simulink library "Wheels_Driver_VehDyn_Lib"  (R2018a)
settings: Solver=VariableStepAuto  StartTime=0.0  StopTime=10.0  RelTol=1e-3
undefined symbols (not defined in the file): I, Kbr, P, vehicleMass
libraries: autolibshared x3, simulink x1
(part 1 of 3)
settings Model: Creator=emarquez  LastModifiedBy=emarquez
settings CodeAppCC: StateflowObjectComments=on

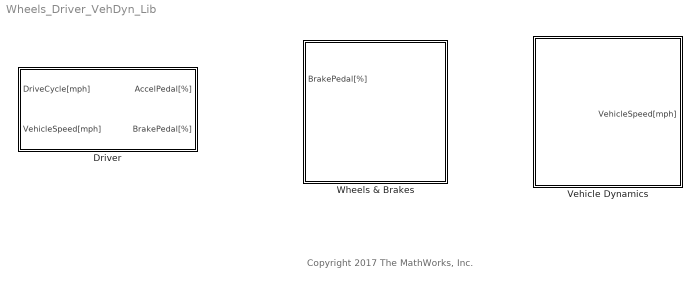
== system Wheels_Driver_VehDyn_Lib ==
  note: Copyright 2017 The MathWorks, Inc.
  Driver : Subsystem
  Vehicle Dynamics : Subsystem
  Wheels & Brakes : Subsystem

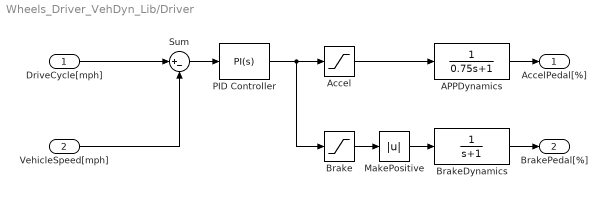
== system Wheels_Driver_VehDyn_Lib/Driver ==
  " DriveCycle[mph]" : Inport
  VehicleSpeed[mph] : Inport  Port=2
  APPDynamics : TransferFcn  Denominator=[0.75 1]
  Accel : Saturate  UpperLimit=100  LowerLimit=0
  Brake : Saturate  UpperLimit=0  LowerLimit=-100
  BrakeDynamics : TransferFcn  Denominator=[1 1]
  MakePositive : Abs
  PID Controller : simulink/Continuous/PID Controller  Controller=PI  TimeDomain=Continuous-time  SampleTime=-1  IntegratorMethod=Forward Euler  FilterMethod=Forward Euler  Form=Parallel  UseFilter=on  ControllerParametersSource=internal  P=P  I=I  D=0  N=100  InitialConditionSource=internal  InitialConditionForIntegrator=0  InitialConditionForFilter=0  ExternalReset=none  LimitOutput=on  UpperSaturationLimit=100  LowerSaturationLimit=-100  LinearizeAsGain=on  AntiWindupMode=none  Kb=1  TrackingMode=off  Kt=1  PParamMin=[]  PParamMax=[]  IParamMin=[]  IParamMax=[]  DParamMin=[]  DParamMax=[]  NParamMin=[]  NParamMax=[]  KbParamMin=[]  KbParamMax=[]  KtParamMin=[]  KtParamMax=[]  POutMin=[]  POutMax=[]  IOutMin=[]  IOutMax=[]  DOutMin=[]  DOutMax=[]  NOutMin=[]  NOutMax=[]  KbOutMin=[]  KbOutMax=[]  KtOutMin=[]  KtOutMax=[]  IntegratorOutMin=[]  IntegratorOutMax=[]  FilterOutMin=[]  FilterOutMax=[]  SumOutMin=[]  SumOutMax=[]  SumI1OutMin=[]  SumI1OutMax=[]  SumI2OutMin=[]  SumI2OutMax=[]  SumI3OutMin=[]  SumI3OutMax=[]  SumDOutMin=[]  SumDOutMax=[]  SaturationOutMin=[]  SaturationOutMax=[]  IntegratorContinuousStateAttributes=''  IntegratorStateMustResolveToSignalObject=off  IntegratorRTWStateStorageClass=Auto  FilterContinuousStateAttributes=''  FilterStateMustResolveToSignalObject=off  FilterRTWStateStorageClass=Auto  DifferentiatorICPrevScaledInput=0  DifferentiatorOutMin=[]  DifferentiatorOutMax=[]  InitialConditionSetting=State (most efficient)  FilterDiffOutCoefMin=[]  FilterDiffOutCoefMax=[]  SumDenOutMin=[]  SumDenOutMax=[]  SumNumOutMin=[]  SumNumOutMax=[]  ReciprocalOutMin=[]  ReciprocalOutMax=[]  DivideOutMin=[]  DivideOutMax=[]  TunerSelectOption=Transfer Function Based (PID Tuner App)
  Sum : Sum  Inputs=|+-
  AccelPedal[%] : Outport
  BrakePedal[%] : Outport  Port=2
  wires:
  APPDynamics/1 -> AccelPedal[%]/1
  Accel/1 -> APPDynamics/1
  Brake/1 -> MakePositive/1
  Sum/1 -> PID Controller/1
  PID Controller/1 -> Brake/1, Accel/1
  VehicleSpeed[mph]/1 -> Sum/2
  " DriveCycle[mph]"/1 -> Sum/1
  BrakeDynamics/1 -> BrakePedal[%]/1
  MakePositive/1 -> BrakeDynamics/1

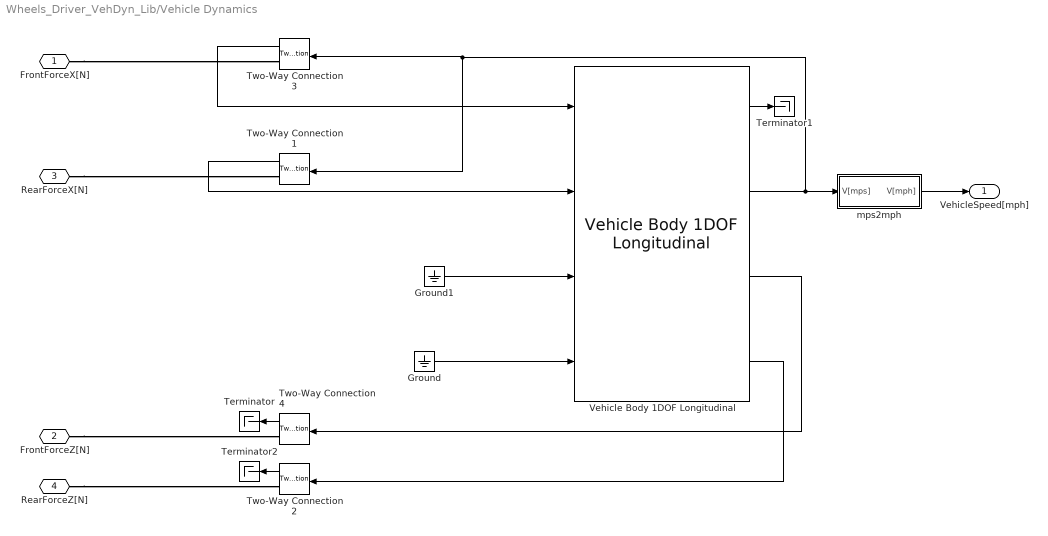
== system Wheels_Driver_VehDyn_Lib/Vehicle Dynamics ==
  Ground : Ground
  Ground1 : Ground
  Terminator : Terminator
  Terminator1 : Terminator
  Terminator2 : Terminator
  Two-Way Connection{1..4} (4 alike) : TwoWayConnection
  Vehicle Body 1DOF Longitudinal : autolibshared/Vehicle Body 1DOF Longitudinal  VariantControl=SL  NF=2  NR=2  m=vehicleMass  a=1.4  b=1.8  h=.35  Cd=.3  Af=4  x_o=0  xdot_o=0  Pabs=101325  T=273  g=9.81
      settings: SourceProductName=Powertrain Blockset  SourceProductBaseCode=PW
  mps2mph : Subsystem
  FrontForceX[N] : PMIOPort  Side=Left
  FrontForceZ[N] : PMIOPort  Port=2  Side=Left
  RearForceX[N] : PMIOPort  Port=3  Side=Left
  RearForceZ[N] : PMIOPort  Port=4  Side=Left
  VehicleSpeed[mph] : Outport
  wires:
  mps2mph/1(V[mph]) -> VehicleSpeed[mph]/1
  Two-Way Connection2/1 -> Terminator2/1
  Two-Way Connection4/1 -> Terminator/1
  Two-Way Connection1/1 -> Vehicle Body 1DOF Longitudinal/2
  Two-Way Connection3/1 -> Vehicle Body 1DOF Longitudinal/1
  Vehicle Body 1DOF Longitudinal/4 -> Two-Way Connection2/1
  Vehicle Body 1DOF Longitudinal/3 -> Two-Way Connection4/1
  Vehicle Body 1DOF Longitudinal/1 -> Terminator1/1
  Vehicle Body 1DOF Longitudinal/2 -> mps2mph/1(V[mps]), Two-Way Connection3/1, Two-Way Connection1/1
  Ground/1 -> Vehicle Body 1DOF Longitudinal/4
  Ground1/1 -> Vehicle Body 1DOF Longitudinal/3
  connections:
  RearForceZ[N]/RConn1 -- Two-Way Connection2/RConn1
  RearForceX[N]/RConn1 -- Two-Way Connection1/RConn1
  FrontForceZ[N]/RConn1 -- Two-Way Connection4/RConn1
  FrontForceX[N]/RConn1 -- Two-Way Connection3/RConn1
